simulink model "IMUFusionSimulinkModel_Android"  (R2020a)
settings: Solver=FixedStepDiscrete  StartTime=0.0  StopTime=30  RelTol=1e-3
model workspace (MAT data in the model file):
  SampleRate = 100
libraries: androidsensorlib x2, mspfiltlib x1, mspsensorlib x1, simulink_extras x1
settings Model: Creator=The MathWorks, Inc.  LastModifiedBy=horia
settings OptimizationCC: EnhancedBackFolding=on  PassReuseOutputArgsAs=Individual arguments  ZeroExternalMemoryAtStartup=off  ZeroInternalMemoryAtStartup=off  MaxStackSize=64  OptimizeBlockOrder=speed  DifferentSizesBufferReuse=on  OptimizationCustomize=off  EfficientTunableParamExpr=on
settings DebuggingCC: ParameterTunabilityLossMsg=error
settings HardwareCC: ProdBitPerPointer=32  ProdBitPerSizeT=32  ProdBitPerPtrDiffT=32  ProdLargestAtomicInteger=Long  ProdLargestAtomicFloat=Double  ProdWordSize=32  ProdHWDeviceType=ARM Compatible->ARM Cortex  UseEmbeddedCoderFeatures=off  UseSimulinkCoderFeatures=off
settings SFSimCC: MATLABDynamicMemAlloc=off
settings RTWCC: SystemTargetFile=ert.tlc  HardwareBoard=Android Device  TemplateMakefile=ert_default_tmf  RTWVerbose=off  Toolchain=Android SDK/NDK Tools
settings CodeAppCC: ForceParamTrailComments=on  IgnoreCustomStorageClasses=off  OperatorAnnotations=on  SimulinkDataObjDesc=on  SFDataObjDesc=on  InsertBlockDesc=on
settings ERTTargetCC: SupportNonInlinedSFcns=on

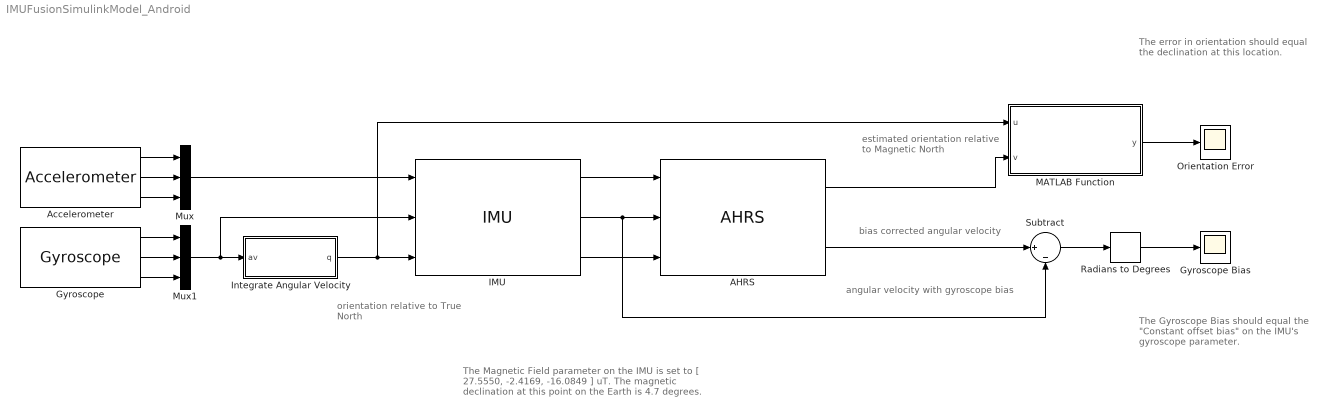
== system IMUFusionSimulinkModel_Android ==
  note: The Magnetic Field parameter on the IMU is set to
      | [ 27.5550, -2.4169, -16.0849 ] uT.
      |
      | The magnetic declination at this point
      | on the Earth is  4.7 degrees.
  note: The Gyroscope Bias should
      | equal the "Constant offset bias"
      | on the IMU's gyroscope parameter.
  note: angular velocity with gyroscope bias
  note: bias corrected angular velocity
  note: The error in orientation should
      | equal the declination at this location.
  note: estimated orientation
      | relative to Magnetic North
  note: orientation relative
      | to True North
  AHRS : mspfiltlib/AHRS  DispRefFrame=NED  DecimationFactor=1  InitialProcessNoise=ahrsfilter.defaultProcessNoise  OrientationFormat=quaternion  SimulateUsing=Code generation  AccelerometerNoise=0.0001924722  GyroscopeNoise=9.1385e-5  MagnetometerNoise=0.1  GyroscopeDriftNoise=3.0462e-13  LinearAccelerationNoise=0.0096236100000000012  MagneticDisturbanceNoise=0.5  LinearAccelerationDecayFactor=0.5  MagneticDisturbanceDecayFactor=0.5  ExpectedMagneticFieldStrength=50
      settings: SourceProductBaseCode=TF,NV
  Accelerometer : androidsensorlib/Accelerometer  OutputVector=off  SampleTime=1/SampleRate  BlockPlatform=Android
      settings: SourceProductBaseCode=ANDROID
  Gyroscope : androidsensorlib/Gyroscope  OutputVector=off  SampleTime=1/SampleRate  BlockPlatform=Android
      settings: SourceProductBaseCode=ANDROID
  Gyroscope Bias : Scope
  IMU : mspsensorlib/IMU  DispRefFrame=NED  Temperature=25  MagneticFieldNED=[ 27.5550, -2.4169, -16.0849 ]  MagneticFieldENU=[ -2.4169, 27.5550, 16.0849 ]  SeedDouble=67  SimulateUsing=Code generation  AccelParamsMeasurementRange=19.613  AccelParamsResolution=0.0023928  AccelParamsConstantBias=[0.19 0.19 0.19]  AccelParamsAxesMisalignment=[0 0 0]  AccelParamsNoiseDensity=[0.0012356 0.0012356 0.0012356]  AccelParamsBiasInstability=[0 0 0]  AccelParamsRandomWalk=[0 0 0]  AccelParamsTemperatureBias=[0 0 0]  AccelParamsTemperatureScaleFactor=[0 0 0]  GyroParamsMeasurementRange=4.3633  GyroParamsResolution=0.0011  GyroParamsConstantBias=[0.0545 0.0545 0.0545]  GyroParamsAxesMisalignment=1.5  GyroParamsAccelerationBias=[0 0 0]  GyroParamsNoiseDensity=[0.00043633 0.00043633 0.00043633]  GyroParamsBiasInstability=[0 0 0]  GyroParamsRandomWalk=[0 0 0]  GyroParamsTemperatureBias=[0 0 0]  GyroParamsTemperatureScaleFactor=[0 0 0]  MagParamsMeasurementRange=1000  MagParamsResolution=0.1  MagParamsConstantBias=0  MagParamsAxesMisalignment=[0 0 0]  MagParamsNoiseDensity=[0.0424 0.0424 0.0424]  MagParamsBiasInstability=[0 0 0]  MagParamsRandomWalk=[0 0 0]  MagParamsTemperatureBias=[0 0 0]  MagParamsTemperatureScaleFactor=[0 0 0]
      settings: SourceProductBaseCode=TF,NV
  Integrate Angular Velocity : MATLAB Function  TreatAsAtomicUnit=on  mask{rate=SampleRate}
      mask prompts: rate "Sample Rate"
  MATLAB Function : MATLAB Function  TreatAsAtomicUnit=on
  Mux : Mux  Inputs=3
  Mux1 : Mux  Inputs=3
  Orientation Error : Scope
  Radians to Degrees : simulink_extras/Transformations/Radians to Degrees
  Subtract : Sum  Inputs=||+|-
  wires:
  IMU/1 -> AHRS/1
  IMU/2 -> Subtract/2, AHRS/2
  IMU/3 -> AHRS/3
  Mux1/1 -> IMU/2, Integrate Angular Velocity/1(av)
  Integrate Angular Velocity/1(q) -> MATLAB Function/1(u), IMU/3
  AHRS/1 -> MATLAB Function/2(v)
  AHRS/2 -> Subtract/1
  MATLAB Function/1(y) -> Orientation Error/1
  Subtract/1 -> Radians to Degrees/1
  Radians to Degrees/1 -> Gyroscope Bias/1
  Accelerometer/1 -> Mux/1
  Accelerometer/2 -> Mux/2
  Accelerometer/3 -> Mux/3
  Mux/1 -> IMU/1
  Gyroscope/1 -> Mux1/1
  Gyroscope/2 -> Mux1/2
  Gyroscope/3 -> Mux1/3

== matlab function IMUFusionSimulinkModel_Android/Integrate Angular Velocity ==
  data: av input; q output; rate parameter
function q = integrateAngVel(av, rate)
%INTEGRATEANGVEL Integrate angular velocity to a quaternion
%  Treat Angular Velocity as an incremental rotation vector.

%   Copyright 2019 The MathWorks, Inc.   

persistent orient
if isempty(orient)
    % Initial orientation is the identity quaternion.
    orient = cast(quaternion(1,0,0,0), 'like', av);
end

% Convert angular velocity to a rotation vector.
rv = quaternion(av*(1/rate), 'rotvec');
orient = rv * orient;
q = compact(orient);

== matlab function IMUFusionSimulinkModel_Android/MATLAB Function ==
  data: u input; y output; v input
function y = orientationError(u,v)
%ORIENTATIONERROR Compute the quaternion distance in degrees

%   Copyright 2019 The MathWorks, Inc.   

y = rad2deg(dist(quaternion(u), quaternion(v)));
